simulink model "sampleModel1621"  (R2023a)
settings: Solver=VariableStepAuto  StartTime=0.0  StopTime=10.0  RelTol=1e-3
libraries: hdlsllib x4, simulink x1
settings Model: Creator=user1  LastModifiedBy=user1

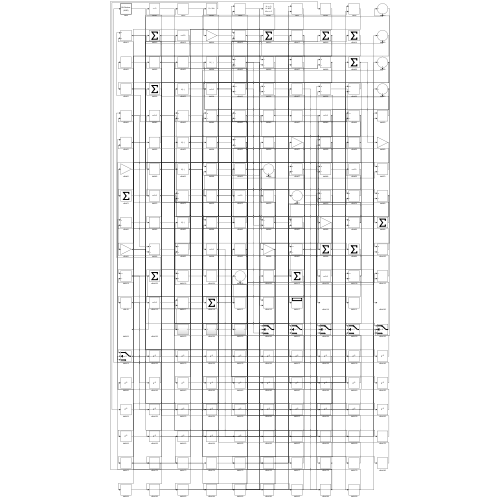
[thumbnail: Simulink's stored preview of the top-level diagram]
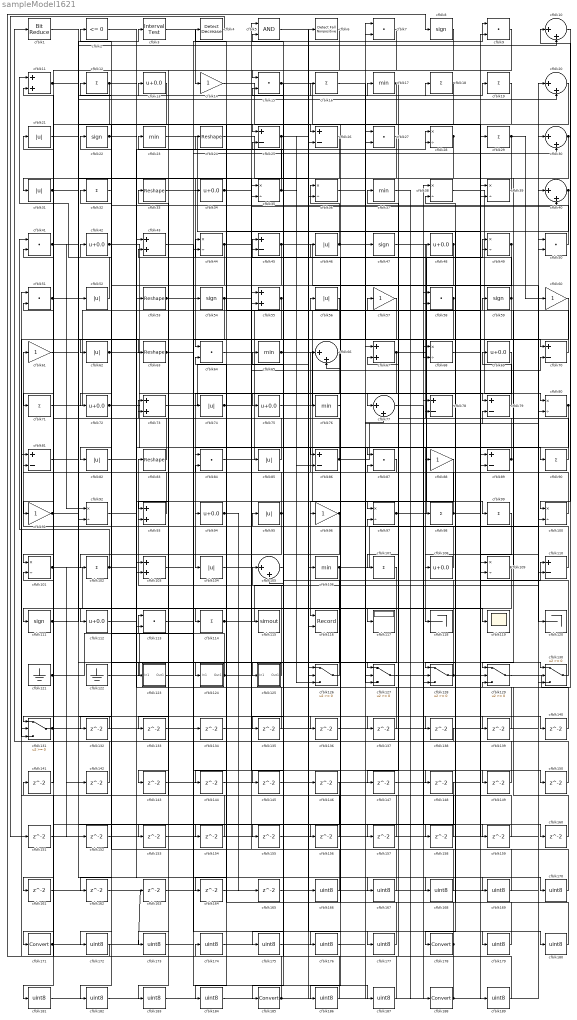
== system sampleModel1621 ==
  cfblk1 : hdlsllib/Logic and Bit Operations/Bit Reduce  mode=AND
  cfblk{10,20,30,40,66,77,105} (7 alike) : Sum  Inputs=|++
  cfblk{28,35..36,38..39,44,49,68,80,92,97,100..101,109} (14 alike) : Product  Inputs=*/  RndMeth=Zero  SaturateOnIntegerOverflow=on
  cfblk{12,16,18..19,29,32,71,90,98..99,102,107,114} (13 alike) : Sum  Inputs=+
  cfblk{11,43,55,67,73,93,103} (7 alike) : Sum
  cfblk{21,31,46,52,56,62,74,82,85,95,104} (11 alike) : Abs  SaturateOnIntegerOverflow=off
  cfblk{17,23,37,65,76,106} (6 alike) : MinMax
  cfblk{13,34,42,48,69,72,75,94,108,112} (10 alike) : Bias  Bias=0.0  SaturateOnIntegerOverflow=off
  cfblk{25..26,45,70,78..79,81,86,89,110} (10 alike) : Sum  Inputs=+-
  cfblk{8,22,47,54,59,111} (6 alike) : Signum
  cfblk{7,9,15,27,41,50..51,58,64,84,87,113} (12 alike) : DotProduct  OutDataTypeStr=Inherit: Inherit via internal rule
  cfblk115 : ToWorkspace  VariableName=simout  SaveFormat=Timeseries  SampleTime=-1
  cfblk116 : Record  FileSettingsInternal="{\"entries\":[{\"content\":{\"excelSettings\":{\"content\":{},\"type\":\"Streamout.ExcelSettings\"}},\"type\":\"Streamout.FileSettingStorage\",\"uuid\":\"\"}],\"packageUris\":[\"http:\\/\\/schema.mathworks.com\\/mf0\\/streamout_blocks\\/R2020a\"],\"version\":\"1.0\"}"  Layout=[1 1]  SignalsInternal="{\"entries\":[{\"content\":{\"signals\":[{\"content\":{\"blockPath\":[],\"dimensions\":[1],\"domain\":\"\",\"lineColor\":\"#a2142f\",\"plots\":[1],\"port\":1,\"signalID\":2341,\"signalName\":\"XY Graph:1\"},\"type\":\"RecordBlkView.Signal\",\"uuid\":\"\"},{\"content\":{\"blockPath\":[],\"dimensions\":[1],\"domain\":\"\",\"lineColor\":\"#139fff\",\"plots\":[1],\"port\":2,\"signalID\":2344,\"signalName\":\"XY Graph:2\"},\"type\":\"RecordBlkView.Signal\",\"uuid\":\"\"}]},\"type\":\"RecordBlkView.InputSignals\",\"uuid\":\"\"}],\"packageUris\":[\"http:\\/\\/schema.mathworks.com\\/mf0\\/streamout_blocks\\/R2020a\"],\"version\":\"1.0\"}"  VisualizationBindings="{\"xyplotplugin\":{\"info\":[{\"series\":[{\"bindingParametersList\":[{\"parameter\":\"X-Axis\",\"signalID\":2341,\"signalName\":\"XY Graph:1\"},{\"parameter\":\"Y-Axis\",\"signalID\":2344,\"signalName\":\"XY Graph:2\"}],\"seriesID\":35827}],\"subplotID\":1}]}}"  CompatibilityTag=XY  st=-1
  cfblk117 : Display
  cfblk118 : Terminator
  cfblk119 : Scope
  cfblk120 : Terminator
  cfblk121 : Ground
  cfblk122 : Ground
  cfblk123 : Subsystem
      settings: LibrarySourceBlock=|
      | hdlsllib/Ports &
      | Subsystems/Subsystem
  cfblk124 : Subsystem
      settings: LibrarySourceBlock=|
      | hdlsllib/Ports &
      | Subsystems/Subsystem
  cfblk125 : Subsystem
      settings: LibrarySourceBlock=|
      | hdlsllib/Ports &
      | Subsystems/Subsystem
  cfblk{126..131} (6 alike) : Switch  SaturateOnIntegerOverflow=off  InputSameDT=off
  cfblk{132..165} (34 alike) : Delay  SampleTime=1
  cfblk{14,57,60..61,88,91,96} (7 alike) : Gain
  cfblk{166..170,172..177,179..184,186..187,189} (20 alike) : DataTypeConversion  OutDataTypeStr=uint8  SaturateOnIntegerOverflow=off  RndMeth=Floor
  cfblk{171,178,185,188} (4 alike) : DataTypeConversion  SaturateOnIntegerOverflow=off  RndMeth=Floor
  cfblk2 : hdlsllib/Logic and Bit Operations/Compare To Zero  relop=<=  OutDataTypeStr=boolean
  cfblk{24,33,53,63,83} (5 alike) : Reshape
  cfblk3 : hdlsllib/Logic and Bit Operations/Interval Test  IntervalClosedRight=on  uplimit=0.5  IntervalClosedLeft=on  lowlimit=-0.5  OutDataTypeStr=boolean
  cfblk4 : simulink/Logic and Bit Operations/Detect Decrease  vinit=0.0  OutDataTypeStr=boolean
      settings: LibrarySourceBlock=|
      | hdlsllib/Logic and Bit
      | Operations/Detect
      | Decrease
  cfblk5 : Logic  AllPortsSameDT=off  OutDataTypeStr=boolean
  cfblk6 : hdlsllib/Logic and Bit Operations/Detect Fall Nonpositive  vinit=0  OutDataTypeStr=boolean
  wires:
  cfblk34/1 -> cfblk148/1, cfblk149/1
  cfblk27/1 -> cfblk64/1
  cfblk38/1 -> cfblk80/1
  cfblk39/1 -> cfblk31/1
  cfblk14/1 -> cfblk26/1
  cfblk46/1 -> cfblk36/1, cfblk19/1
  cfblk121/1 -> cfblk113/1, cfblk101/2
  cfblk130/1 -> cfblk45/1
  cfblk84/1 -> cfblk56/1
  cfblk47/1 -> cfblk90/1
  cfblk29/1 -> cfblk75/1, cfblk60/1
  cfblk97/1 -> cfblk49/1, cfblk159/1
  cfblk108/1 -> cfblk61/1
  cfblk78/1 -> cfblk178/1
  cfblk42/1 -> cfblk77/1, cfblk28/1
  cfblk41/1 -> cfblk52/1, cfblk10/2
  cfblk125/1(Out1) -> cfblk83/1
  cfblk69/1 -> cfblk104/1
  cfblk129/1 -> cfblk10/1
  cfblk52/1 -> cfblk11/1
  cfblk22/1 -> cfblk103/1, cfblk98/1
  cfblk26/1 -> cfblk124/1(In1)
  cfblk17/1 -> cfblk34/1, cfblk147/1
  cfblk71/1 -> cfblk29/1
  cfblk131/1 -> cfblk27/2, cfblk167/1
  cfblk44/1 -> cfblk17/1, cfblk112/1, cfblk4/1
  cfblk62/1 -> cfblk118/1, cfblk87/1
  cfblk30/1 -> cfblk129/1, cfblk117/1
  cfblk8/1 -> cfblk171/1
  cfblk94/1 -> cfblk164/1, cfblk165/1
  cfblk67/1 -> cfblk99/1, cfblk155/1
  cfblk20/1 -> cfblk62/1
  cfblk73/1 -> cfblk26/2
  cfblk10/1 -> cfblk100/1
  cfblk75/1 -> cfblk39/1
  cfblk89/1 -> cfblk48/1, cfblk67/2
  cfblk91/1 -> cfblk136/1, cfblk137/1, cfblk138/1
  cfblk74/1 -> cfblk85/1, cfblk16/1
  cfblk65/1 -> cfblk97/1, cfblk160/1
  cfblk24/1 -> cfblk36/2
  cfblk128/1 -> cfblk73/1, cfblk110/1
  cfblk86/1 -> cfblk33/1, cfblk40/1
  cfblk18/1 -> cfblk96/1, cfblk143/1
  cfblk16/1 -> cfblk47/1
  cfblk93/1 -> cfblk12/1
  cfblk51/1 -> cfblk3/1, cfblk92/1
  cfblk70/1 -> cfblk44/1
  cfblk45/1 -> cfblk120/1, cfblk123/1(In1)
  cfblk82/1 -> cfblk103/2
  cfblk79/1 -> cfblk69/1
  cfblk72/1 -> cfblk88/1, cfblk86/1
  cfblk66/1 -> cfblk74/1
  cfblk98/1 -> cfblk65/1, cfblk110/2
  cfblk109/1 -> cfblk111/1, cfblk59/1
  cfblk88/1 -> cfblk116/1
  cfblk99/1 -> cfblk128/1
  cfblk19/1 -> cfblk114/1
  cfblk55/1 -> cfblk93/1, cfblk71/1
  cfblk80/1 -> cfblk94/1, cfblk127/3
  cfblk114/1 -> cfblk80/2, cfblk70/2, cfblk84/2
  cfblk11/1 -> cfblk20/2, cfblk25/1
  cfblk124/1(Out1) -> cfblk32/1, cfblk40/2
  cfblk50/1 -> cfblk22/1
  cfblk33/1 -> cfblk109/2
  cfblk1/1 -> cfblk35/2
  cfblk36/1 -> cfblk70/1
  cfblk40/1 -> cfblk108/1, cfblk154/1
  cfblk105/1 -> cfblk185/1
  cfblk102/1 -> cfblk41/1, cfblk128/2
  cfblk83/1 -> cfblk42/1
  cfblk54/1 -> cfblk49/2, cfblk162/1
  cfblk63/1 -> cfblk156/1, cfblk177/1, cfblk179/1
  cfblk25/1 -> cfblk79/1, cfblk86/2, cfblk28/2, cfblk92/2
  cfblk61/1 -> cfblk13/1
  cfblk95/1 -> cfblk102/1, cfblk51/2, cfblk25/2, cfblk132/1
  cfblk104/1 -> cfblk57/1
  cfblk113/1 -> cfblk9/1
  cfblk111/1 -> cfblk18/1, cfblk142/1
  cfblk100/1 -> cfblk66/1
  cfblk21/1 -> cfblk113/2
  cfblk37/1 -> cfblk188/1
  cfblk32/1 -> cfblk72/1
  cfblk15/1 -> cfblk89/2, cfblk175/1
  cfblk3/1 -> cfblk14/1
  cfblk85/1 -> cfblk21/1
  cfblk106/1 -> cfblk50/1, cfblk79/2, cfblk172/1
  cfblk13/1 -> cfblk101/1
  cfblk87/1 -> cfblk81/2
  cfblk53/1 -> cfblk119/1, cfblk150/1
  cfblk123/1(Out1) -> cfblk30/2
  cfblk31/1 -> cfblk63/1, cfblk157/1
  cfblk23/1 -> cfblk115/1
  cfblk58/1 -> cfblk131/3, cfblk66/2
  cfblk112/1 -> cfblk53/1
  cfblk122/1 -> cfblk44/2
  cfblk28/1 -> cfblk82/1, cfblk84/1
  cfblk126/1 -> cfblk43/2
  cfblk64/1 -> cfblk127/1
  cfblk96/1 -> cfblk125/1(In1), cfblk145/1
  cfblk12/1 -> cfblk91/1, cfblk127/2
  cfblk81/1 -> cfblk130/1
  cfblk110/1 -> cfblk93/2
  cfblk49/1 -> cfblk107/1, cfblk55/2
  cfblk48/1 -> cfblk133/1, cfblk184/1
  cfblk35/1 -> cfblk23/1, cfblk126/3
  cfblk9/1 -> cfblk15/1
  cfblk43/1 -> cfblk68/2
  cfblk59/1 -> cfblk24/1, cfblk182/1
  cfblk90/1 -> cfblk38/2
  cfblk101/1 -> cfblk116/2, cfblk152/1, cfblk153/1
  cfblk132/1 -> cfblk131/1
  cfblk103/1 -> cfblk134/1
  cfblk134/1 -> cfblk30/1
  cfblk107/1 -> cfblk135/1
  cfblk135/1 -> cfblk43/1
  cfblk136/1 -> cfblk68/1
  cfblk137/1 -> cfblk55/1
  cfblk138/1 -> cfblk1/1
  cfblk127/1 -> cfblk139/1
  cfblk139/1 -> cfblk126/2
  cfblk77/1 -> cfblk140/1
  cfblk140/1 -> cfblk35/1
  cfblk141/1 -> cfblk41/2
  cfblk142/1 -> cfblk11/2
  cfblk143/1 -> cfblk39/2
  cfblk56/1 -> cfblk144/1
  cfblk144/1 -> cfblk9/2
  cfblk145/1 -> cfblk129/2
  cfblk147/1 -> cfblk109/1
  cfblk149/1 -> cfblk97/2
  cfblk150/1 -> cfblk131/2
  cfblk4/1 -> cfblk151/1
  cfblk151/1 -> cfblk89/1
  cfblk152/1 -> cfblk100/2
  cfblk153/1 -> cfblk130/3
  cfblk154/1 -> cfblk73/2
  cfblk156/1 -> cfblk45/2
  cfblk157/1 -> cfblk15/2
  cfblk60/1 -> cfblk158/1
  cfblk158/1 -> cfblk81/1
  cfblk159/1 -> cfblk87/2
  cfblk160/1 -> cfblk129/3
  cfblk57/1 -> cfblk161/1
  cfblk161/1 -> cfblk20/1
  cfblk162/1 -> cfblk126/1
  cfblk163/1 -> cfblk58/2
  cfblk164/1 -> cfblk38/1
  cfblk165/1 -> cfblk130/2
  cfblk5/1 -> cfblk166/1
  cfblk166/1 -> cfblk95/1
  cfblk167/1 -> cfblk5/1
  cfblk133/1 -> cfblk168/1
  cfblk168/1 -> cfblk5/2
  cfblk2/1 -> cfblk169/1
  cfblk169/1 -> cfblk46/1
  cfblk92/1 -> cfblk170/1
  cfblk170/1 -> cfblk2/1
  cfblk171/1 -> cfblk163/1, cfblk54/1
  cfblk172/1 -> cfblk8/1
  cfblk7/1 -> cfblk173/1
  cfblk174/1 -> cfblk7/1
  cfblk175/1 -> cfblk7/2
  cfblk76/1 -> cfblk176/1
  cfblk176/1 -> cfblk27/1
  cfblk177/1 -> cfblk76/1
  cfblk178/1 -> cfblk174/1, cfblk64/2
  cfblk179/1 -> cfblk78/1
  cfblk155/1 -> cfblk180/1
  cfblk180/1 -> cfblk78/2
  cfblk146/1 -> cfblk181/1
  cfblk181/1 -> cfblk50/2
  cfblk182/1 -> cfblk146/1
  cfblk6/1 -> cfblk183/1
  cfblk183/1 -> cfblk106/1
  cfblk184/1 -> cfblk6/1
  cfblk185/1 -> cfblk141/1, cfblk128/3, cfblk67/1, cfblk77/2
  cfblk148/1 -> cfblk186/1
  cfblk186/1 -> cfblk105/1
  cfblk173/1 -> cfblk187/1
  cfblk187/1 -> cfblk105/2
  cfblk188/1 -> cfblk51/1, cfblk58/1
  cfblk68/1 -> cfblk189/1
  cfblk189/1 -> cfblk37/1

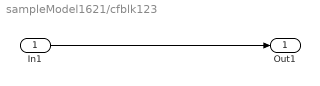
== system sampleModel1621/cfblk123 ==
  In1 : Inport
  Out1 : Outport
  wires:
  In1/1 -> Out1/1

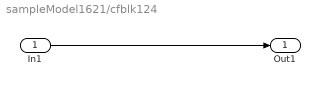
== system sampleModel1621/cfblk124 ==
  In1 : Inport
  Out1 : Outport
  wires:
  In1/1 -> Out1/1

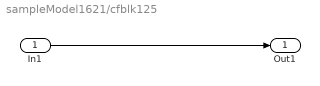
== system sampleModel1621/cfblk125 ==
  In1 : Inport
  Out1 : Outport
  wires:
  In1/1 -> Out1/1
